simulink model "prop_thrust"  (R2013b)
settings: Solver=FixedStepDiscrete  StartTime=0.0  StopTime=2100  FixedStep=1  RelTol=1e-3
undefined symbols (not defined in the file): DiscIntNeverNeededParam
libraries: simulink x1
settings Model: Creator=pkarplus  LastModifiedBy=pkarplus

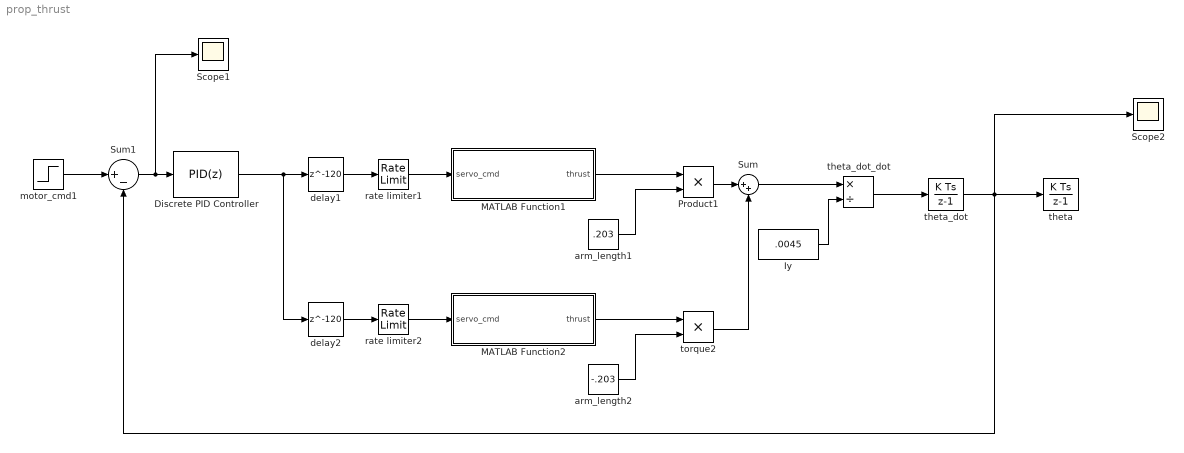
== system prop_thrust ==
  Discrete PID Controller : simulink/Continuous/PID Controller  Controller=PID  TimeDomain=Discrete-time  SampleTime=1  IntegratorMethod=Forward Euler  FilterMethod=Forward Euler  Form=Parallel  P=.001  I=.0001  D=.0001  N=100  InitialConditionSource=internal  InitialConditionForIntegrator=0  InitialConditionForFilter=0  ExternalReset=none  LimitOutput=on  UpperSaturationLimit=100  LowerSaturationLimit=-100  LinearizeAsGain=off  AntiWindupMode=clamping  Kb=1  TrackingMode=off  Kt=1  PParamMin=[]  PParamMax=[]  IParamMin=[]  IParamMax=[]  DParamMin=[]  DParamMax=[]  NParamMin=[]  NParamMax=[]  KbParamMin=[]  KbParamMax=[]  KtParamMin=[]  KtParamMax=[]  POutMin=[]  POutMax=[]  IOutMin=[]  IOutMax=[]  DOutMin=[]  DOutMax=[]  NOutMin=[]  NOutMax=[]  KbOutMin=[]  KbOutMax=[]  KtOutMin=[]  KtOutMax=[]  IntegratorOutMin=[]  IntegratorOutMax=[]  FilterOutMin=[]  FilterOutMax=[]  SumOutMin=[]  SumOutMax=[]  SumI1OutMin=[]  SumI1OutMax=[]  SumI2OutMin=[]  SumI2OutMax=[]  SumI3OutMin=[]  SumI3OutMax=[]  SumDOutMin=[]  SumDOutMax=[]  SaturationOutMin=[]  SaturationOutMax=[]  IntegratorContinuousStateAttributes=''  IntegratorStateMustResolveToSignalObject=off  IntegratorRTWStateStorageClass=Auto  FilterContinuousStateAttributes=''  FilterStateMustResolveToSignalObject=off  FilterRTWStateStorageClass=Auto
  Iy : Constant  Value=.0045
  MATLAB Function1 : MATLAB Function  TreatAsAtomicUnit=on
  MATLAB Function2 : MATLAB Function  TreatAsAtomicUnit=on
  Product1 : Product
  Scope1 : Scope
  Scope2 : Scope
      settings: SaveName=ScopeData2
  Sum : Sum  Inputs=|++
  Sum1 : Sum  Inputs=|+-
  arm_length1 : Constant  Value=.203
  arm_length2 : Constant  Value=-.203
  delay1 : Delay  DelayLength=120  InitialCondition=0  SampleTime=1
  delay2 : Delay  DelayLength=120  InitialCondition=0  SampleTime=1
  motor_cmd1 : Step  Time=1000  After=100  SampleTime=0
  rate limiter1 : RateLimiter  RisingSlewLimit=1000/300  SampleTimeMode=inherited
  rate limiter2 : RateLimiter  RisingSlewLimit=1000/400  SampleTimeMode=inherited
  theta : DiscreteIntegrator  gainval=1/1000  LimitOutput=on  UpperSaturationLimit=90  LowerSaturationLimit=-90  ICPrevOutput=DiscIntNeverNeededParam  ICPrevScaledInput=DiscIntNeverNeededParam
  theta_dot : DiscreteIntegrator  gainval=1/1000  LimitOutput=on  UpperSaturationLimit=30000  LowerSaturationLimit=-30000  ICPrevOutput=DiscIntNeverNeededParam  ICPrevScaledInput=DiscIntNeverNeededParam
  theta_dot_dot : Product  Inputs=*/
  torque2 : Product
  wires:
  Discrete PID Controller/1 -> delay2/1, delay1/1
  delay2/1 -> rate limiter2/1
  rate limiter2/1 -> MATLAB Function2/1(servo_cmd)
  MATLAB Function2/1(thrust) -> torque2/1
  arm_length2/1 -> torque2/2
  torque2/1 -> Sum/2
  delay1/1 -> rate limiter1/1
  rate limiter1/1 -> MATLAB Function1/1(servo_cmd)
  MATLAB Function1/1(thrust) -> Product1/1
  arm_length1/1 -> Product1/2
  Product1/1 -> Sum/1
  Iy/1 -> theta_dot_dot/2
  Sum/1 -> theta_dot_dot/1
  theta_dot_dot/1 -> theta_dot/1
  theta_dot/1 -> Scope2/1, theta/1, Sum1/2
  motor_cmd1/1 -> Sum1/1
  Sum1/1 -> Scope1/1, Discrete PID Controller/1

== matlab function prop_thrust/MATLAB Function1 ==
  data: servo_cmd input; thrust output
function thrust = prop_thrust(servo_cmd)
%#codegen
Prop_Data = ...
[0	0
1697.14285714286	22
2382.85714285714	42
2682.85714285714	54
3248.57142857143	84
3574.28571428571	102
4122.85714285714	129
4285.71428571429	152
4654.28571428571	167
4868.57142857143	180
5100	215
5640	248
5717.14285714286	267
6214.28571428571	290
6591.42857142857	345
6805.71428571429	385]; % 8045R Propeller  (RPM, Thrust (g))

% Scale to 0-1000 scale for RPM
Prop_Data(:,1) = Prop_Data(:,1)/Prop_Data(end,1)*1000;

% Scale from grams to Newtons
Prop_Data(:,2) = Prop_Data(:,2)*9.81/1000;

thrust = interp1(Prop_Data(:,1),Prop_Data(:,2),servo_cmd);

== matlab function prop_thrust/MATLAB Function2 ==
  data: servo_cmd input; thrust output
function thrust = prop_thrust(servo_cmd)
%#codegen
Prop_Data = ...
[0	0
1697.14285714286	22
2382.85714285714	42
2682.85714285714	54
3248.57142857143	84
3574.28571428571	102
4122.85714285714	129
4285.71428571429	152
4654.28571428571	167
4868.57142857143	180
5100	215
5640	248
5717.14285714286	267
6214.28571428571	290
6591.42857142857	345
6805.71428571429	385]; % 8045R Propeller  (RPM, Thrust (g))

% Scale to 0-1000 scale for RPM
Prop_Data(:,1) = Prop_Data(:,1)/Prop_Data(end,1)*1000;

% Scale from grams to Newtons
Prop_Data(:,2) = Prop_Data(:,2)*9.81/1000;

thrust = interp1(Prop_Data(:,1),Prop_Data(:,2),servo_cmd);
